simulink model "FLC_tracking_comparison_of_quadrotor"  (R2015a)
settings: Solver=ode3  StartTime=0.0  StopTime=10  FixedStep=0.01  RelTol=1e-3
libraries: simulink x9, commnoisgen2 x5, fuzblock x4
settings Model: SimulationMode=accelerator  Creator=user  LastModifiedBy=user
settings OptimizationCC: EfficientMapNaN2IntZero=off
settings HardwareCC: TargetLongLongMode=on  TargetIntDivRoundTo=Zero  TargetEndianess=LittleEndian  TargetHWDeviceType=MATLAB Host  ProdEqTarget=off
settings CodeAppCC: MaxIdLength=128
settings GRTTargetCC: CombineOutputUpdateFcns=off  GRTInterface=on

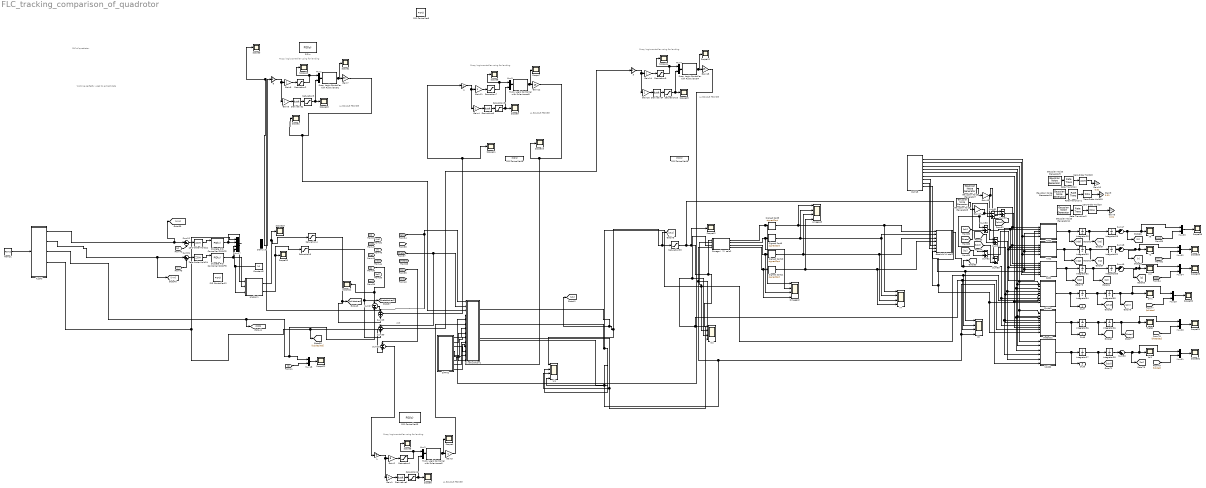
== system FLC_tracking_comparison_of_quadrotor ==
  note: Working perfectly used to extract data
  note: FLC of quadrotor
  note: d25
  note: Fuzzy logic controller using for landing
  note: LA BOUCLE FERMEE
  note: Fuzzy logic controller using for landing
  note: LA BOUCLE FERMEE
  note: Fuzzy logic controller using for landing
  note: LA BOUCLE FERMEE
  note: Fuzzy logic controller using for landing
  note: LA BOUCLE FERMEE
  1 : Gain  Gain=5
  2 : Gain
  3 : Gain
  8 : Gain  Gain=5
  Constant2 : Constant  Value=10
  DATA2 : MATLAB Function  TreatAsAtomicUnit=on
  DATA5 : MATLAB Function  TreatAsAtomicUnit=on
  Demux3 : Demux  Outputs=2
  Derivative{1..4} (4 alike) : Derivative
  Discrete PID Controller (2DOF)2 : simulink/Continuous/PID Controller (2DOF)  Controller=PID  TimeDomain=Discrete-time  SampleTime=0.01  IntegratorMethod=Forward Euler  FilterMethod=Forward Euler  Form=Parallel  UseFilter=on  ControllerParametersSource=internal  P=40  I=10  D=1  N=100  b=1  c=1  InitialConditionSource=internal  InitialConditionForIntegrator=0  InitialConditionForFilter=0  ExternalReset=none  LimitOutput=off  UpperSaturationLimit=inf  LowerSaturationLimit=-inf  LinearizeAsGain=off  AntiWindupMode=none  Kb=1  TrackingMode=off  Kt=1  PParamMin=[]  PParamMax=[]  IParamMin=[]  IParamMax=[]  DParamMin=[]  DParamMax=[]  NParamMin=[]  NParamMax=[]  bParamMin=[]  bParamMax=[]  cParamMin=[]  cParamMax=[]  KbParamMin=[]  KbParamMax=[]  KtParamMin=[]  KtParamMax=[]  POutMin=[]  POutMax=[]  IOutMin=[]  IOutMax=[]  DOutMin=[]  DOutMax=[]  NOutMin=[]  NOutMax=[]  bOutMin=[]  bOutMax=[]  cOutMin=[]  cOutMax=[]  KbOutMin=[]  KbOutMax=[]  KtOutMin=[]  KtOutMax=[]  IntegratorOutMin=[]  IntegratorOutMax=[]  FilterOutMin=[]  FilterOutMax=[]  SumOutMin=[]  SumOutMax=[]  Sum1OutMin=[]  Sum1OutMax=[]  Sum2OutMin=[]  Sum2OutMax=[]  Sum3OutMin=[]  Sum3OutMax=[]  SumI1OutMin=[]  SumI1OutMax=[]  SumI2OutMin=[]  SumI2OutMax=[]  SumI3OutMin=[]  SumI3OutMax=[]  SumDOutMin=[]  SumDOutMax=[]  SaturationOutMin=[]  SaturationOutMax=[]  IntegratorContinuousStateAttributes=''  IntegratorStateMustResolveToSignalObject=off  IntegratorRTWStateStorageClass=Auto  FilterContinuousStateAttributes=''  FilterStateMustResolveToSignalObject=off  FilterRTWStateStorageClass=Auto  DifferentiatorICPrevScaledInput=0  DifferentiatorOutMin=[]  DifferentiatorOutMax=[]
  Discrete PID Controller (2DOF)3 : simulink/Continuous/PID Controller (2DOF)  Controller=PID  TimeDomain=Discrete-time  SampleTime=0.01  IntegratorMethod=Forward Euler  FilterMethod=Forward Euler  Form=Parallel  UseFilter=on  ControllerParametersSource=internal  P=30  I=8  D=2.4  N=100  b=1  c=1  InitialConditionSource=internal  InitialConditionForIntegrator=0  InitialConditionForFilter=0  ExternalReset=none  LimitOutput=off  UpperSaturationLimit=inf  LowerSaturationLimit=-inf  LinearizeAsGain=off  AntiWindupMode=none  Kb=1  TrackingMode=off  Kt=1  PParamMin=[]  PParamMax=[]  IParamMin=[]  IParamMax=[]  DParamMin=[]  DParamMax=[]  NParamMin=[]  NParamMax=[]  bParamMin=[]  bParamMax=[]  cParamMin=[]  cParamMax=[]  KbParamMin=[]  KbParamMax=[]  KtParamMin=[]  KtParamMax=[]  POutMin=[]  POutMax=[]  IOutMin=[]  IOutMax=[]  DOutMin=[]  DOutMax=[]  NOutMin=[]  NOutMax=[]  bOutMin=[]  bOutMax=[]  cOutMin=[]  cOutMax=[]  KbOutMin=[]  KbOutMax=[]  KtOutMin=[]  KtOutMax=[]  IntegratorOutMin=[]  IntegratorOutMax=[]  FilterOutMin=[]  FilterOutMax=[]  SumOutMin=[]  SumOutMax=[]  Sum1OutMin=[]  Sum1OutMax=[]  Sum2OutMin=[]  Sum2OutMax=[]  Sum3OutMin=[]  Sum3OutMax=[]  SumI1OutMin=[]  SumI1OutMax=[]  SumI2OutMin=[]  SumI2OutMax=[]  SumI3OutMin=[]  SumI3OutMax=[]  SumDOutMin=[]  SumDOutMax=[]  SaturationOutMin=[]  SaturationOutMax=[]  IntegratorContinuousStateAttributes=''  IntegratorStateMustResolveToSignalObject=off  IntegratorRTWStateStorageClass=Auto  FilterContinuousStateAttributes=''  FilterStateMustResolveToSignalObject=off  FilterRTWStateStorageClass=Auto  DifferentiatorICPrevScaledInput=0  DifferentiatorOutMin=[]  DifferentiatorOutMax=[]
  Fuzzy Logic Controller with Ruleviewer{1..4} (4 alike) : fuzblock/Fuzzy Logic  Controller  with Ruleviewer  fismatrix=fuzzytrial7  Ts=2
  Gain1 : Gain  Gain=4
  Gain{8..10,13,17} (5 alike) : Gain  Gain=0.01
  Gain{3..6,11,14,16} (7 alike) : Gain
  Gain12 : Gain  Gain=15
  Gain15 : Gain  Gain=15
  Gain2 : Gain  Gain=8
  Gain7 : Gain  Gain=50
  Gaussian Noise Generator10 : commnoisgen2/Gaussian Noise Generator  m=0  d=1  s=41  Ts=3  frameBased=off  sampPerFrame=1  orient=off  outDataType=single
  Gaussian Noise Generator11 : commnoisgen2/Gaussian Noise Generator  m=0  d=1  s=41  Ts=4  frameBased=off  sampPerFrame=1  orient=off  outDataType=single
  Gaussian Noise Generator7 : commnoisgen2/Gaussian Noise Generator  m=0  d=1  s=41  Ts=0.01  frameBased=off  sampPerFrame=1  orient=off  outDataType=double
  Gaussian Noise Generator8 : commnoisgen2/Gaussian Noise Generator  m=0  d=1  s=41  Ts=0.01  frameBased=off  sampPerFrame=1  orient=off  outDataType=double
  Gaussian Noise Generator9 : commnoisgen2/Gaussian Noise Generator  m=0  d=1  s=41  Ts=5  frameBased=off  sampPerFrame=1  orient=off  outDataType=single
  Integrator{25..36} (12 alike) : Integrator
  Mux{1..4,18,29..34} (11 alike) : Mux  Inputs=2
  Mux17 : Mux
  Omega i ^2  calc2 : MATLAB Function  TreatAsAtomicUnit=on
  Omegas2 : Scope  NumInputPorts=4
      settings: YMin=-5~-5~-5~-5  YMax=5~5~5~5  SaveName=ScopeData36
  PID Controller12 : simulink/Continuous/PID Controller  Controller=PID  TimeDomain=Continuous-time  SampleTime=-1  IntegratorMethod=Forward Euler  FilterMethod=Forward Euler  Form=Parallel  UseFilter=on  ControllerParametersSource=internal  P=1.8  I=0.4  D=2.4  N=100  InitialConditionSource=internal  InitialConditionForIntegrator=0  InitialConditionForFilter=0  ExternalReset=none  LimitOutput=off  UpperSaturationLimit=inf  LowerSaturationLimit=-inf  LinearizeAsGain=on  AntiWindupMode=none  Kb=1  TrackingMode=off  Kt=1  PParamMin=[]  PParamMax=[]  IParamMin=[]  IParamMax=[]  DParamMin=[]  DParamMax=[]  NParamMin=[]  NParamMax=[]  KbParamMin=[]  KbParamMax=[]  KtParamMin=[]  KtParamMax=[]  POutMin=[]  POutMax=[]  IOutMin=[]  IOutMax=[]  DOutMin=[]  DOutMax=[]  NOutMin=[]  NOutMax=[]  KbOutMin=[]  KbOutMax=[]  KtOutMin=[]  KtOutMax=[]  IntegratorOutMin=[]  IntegratorOutMax=[]  FilterOutMin=[]  FilterOutMax=[]  SumOutMin=[]  SumOutMax=[]  SumI1OutMin=[]  SumI1OutMax=[]  SumI2OutMin=[]  SumI2OutMax=[]  SumI3OutMin=[]  SumI3OutMax=[]  SumDOutMin=[]  SumDOutMax=[]  SaturationOutMin=[]  SaturationOutMax=[]  IntegratorContinuousStateAttributes=''  IntegratorStateMustResolveToSignalObject=off  IntegratorRTWStateStorageClass=Auto  FilterContinuousStateAttributes=''  FilterStateMustResolveToSignalObject=off  FilterRTWStateStorageClass=Auto  DifferentiatorICPrevScaledInput=0  DifferentiatorOutMin=[]  DifferentiatorOutMax=[]
  PID Controller13 : simulink/Continuous/PID Controller  Controller=PID  TimeDomain=Continuous-time  SampleTime=-1  IntegratorMethod=Forward Euler  FilterMethod=Forward Euler  Form=Parallel  UseFilter=on  ControllerParametersSource=internal  P=4.05643234281984  I=0.70959032661118  D=4.0859309721323  N=476.409993785115  InitialConditionSource=internal  InitialConditionForIntegrator=0  InitialConditionForFilter=0  ExternalReset=none  LimitOutput=off  UpperSaturationLimit=inf  LowerSaturationLimit=-inf  LinearizeAsGain=on  AntiWindupMode=none  Kb=1  TrackingMode=off  Kt=1  PParamMin=[]  PParamMax=[]  IParamMin=[]  IParamMax=[]  DParamMin=[]  DParamMax=[]  NParamMin=[]  NParamMax=[]  KbParamMin=[]  KbParamMax=[]  KtParamMin=[]  KtParamMax=[]  POutMin=[]  POutMax=[]  IOutMin=[]  IOutMax=[]  DOutMin=[]  DOutMax=[]  NOutMin=[]  NOutMax=[]  KbOutMin=[]  KbOutMax=[]  KtOutMin=[]  KtOutMax=[]  IntegratorOutMin=[]  IntegratorOutMax=[]  FilterOutMin=[]  FilterOutMax=[]  SumOutMin=[]  SumOutMax=[]  SumI1OutMin=[]  SumI1OutMax=[]  SumI2OutMin=[]  SumI2OutMax=[]  SumI3OutMin=[]  SumI3OutMax=[]  SumDOutMin=[]  SumDOutMax=[]  SaturationOutMin=[]  SaturationOutMax=[]  IntegratorContinuousStateAttributes=''  IntegratorStateMustResolveToSignalObject=off  IntegratorRTWStateStorageClass=Auto  FilterContinuousStateAttributes=''  FilterStateMustResolveToSignalObject=off  FilterRTWStateStorageClass=Auto  DifferentiatorICPrevScaledInput=0  DifferentiatorOutMin=[]  DifferentiatorOutMax=[]
  PID Controller15 : simulink/Continuous/PID Controller  Controller=PID  TimeDomain=Continuous-time  SampleTime=-1  IntegratorMethod=Forward Euler  FilterMethod=Forward Euler  Form=Parallel  UseFilter=on  ControllerParametersSource=internal  P=11  I=0.2  D=22  N=100  InitialConditionSource=internal  InitialConditionForIntegrator=0  InitialConditionForFilter=0  ExternalReset=none  LimitOutput=off  UpperSaturationLimit=inf  LowerSaturationLimit=-inf  LinearizeAsGain=on  AntiWindupMode=none  Kb=1  TrackingMode=off  Kt=1  PParamMin=[]  PParamMax=[]  IParamMin=[]  IParamMax=[]  DParamMin=[]  DParamMax=[]  NParamMin=[]  NParamMax=[]  KbParamMin=[]  KbParamMax=[]  KtParamMin=[]  KtParamMax=[]  POutMin=[]  POutMax=[]  IOutMin=[]  IOutMax=[]  DOutMin=[]  DOutMax=[]  NOutMin=[]  NOutMax=[]  KbOutMin=[]  KbOutMax=[]  KtOutMin=[]  KtOutMax=[]  IntegratorOutMin=[]  IntegratorOutMax=[]  FilterOutMin=[]  FilterOutMax=[]  SumOutMin=[]  SumOutMax=[]  SumI1OutMin=[]  SumI1OutMax=[]  SumI2OutMin=[]  SumI2OutMax=[]  SumI3OutMin=[]  SumI3OutMax=[]  SumDOutMin=[]  SumDOutMax=[]  SaturationOutMin=[]  SaturationOutMax=[]  IntegratorContinuousStateAttributes=''  IntegratorStateMustResolveToSignalObject=off  IntegratorRTWStateStorageClass=Auto  FilterContinuousStateAttributes=''  FilterStateMustResolveToSignalObject=off  FilterRTWStateStorageClass=Auto  DifferentiatorICPrevScaledInput=0  DifferentiatorOutMin=[]  DifferentiatorOutMax=[]
  PID Controller16 : simulink/Continuous/PID Controller  Controller=PID  TimeDomain=Continuous-time  SampleTime=-1  IntegratorMethod=Forward Euler  FilterMethod=Forward Euler  Form=Parallel  UseFilter=on  ControllerParametersSource=internal  P=12  I=0.2  D=20  N=100  InitialConditionSource=internal  InitialConditionForIntegrator=0  InitialConditionForFilter=0  ExternalReset=none  LimitOutput=off  UpperSaturationLimit=inf  LowerSaturationLimit=-inf  LinearizeAsGain=on  AntiWindupMode=none  Kb=1  TrackingMode=off  Kt=1  PParamMin=[]  PParamMax=[]  IParamMin=[]  IParamMax=[]  DParamMin=[]  DParamMax=[]  NParamMin=[]  NParamMax=[]  KbParamMin=[]  KbParamMax=[]  KtParamMin=[]  KtParamMax=[]  POutMin=[]  POutMax=[]  IOutMin=[]  IOutMax=[]  DOutMin=[]  DOutMax=[]  NOutMin=[]  NOutMax=[]  KbOutMin=[]  KbOutMax=[]  KtOutMin=[]  KtOutMax=[]  IntegratorOutMin=[]  IntegratorOutMax=[]  FilterOutMin=[]  FilterOutMax=[]  SumOutMin=[]  SumOutMax=[]  SumI1OutMin=[]  SumI1OutMax=[]  SumI2OutMin=[]  SumI2OutMax=[]  SumI3OutMin=[]  SumI3OutMax=[]  SumDOutMin=[]  SumDOutMax=[]  SaturationOutMin=[]  SaturationOutMax=[]  IntegratorContinuousStateAttributes=''  IntegratorStateMustResolveToSignalObject=off  IntegratorRTWStateStorageClass=Auto  FilterContinuousStateAttributes=''  FilterStateMustResolveToSignalObject=off  FilterRTWStateStorageClass=Auto  DifferentiatorICPrevScaledInput=0  DifferentiatorOutMin=[]  DifferentiatorOutMax=[]
  PID Controller8 : simulink/Continuous/PID Controller  Controller=PID  TimeDomain=Discrete-time  SampleTime=0.01  IntegratorMethod=Forward Euler  FilterMethod=Forward Euler  Form=Parallel  UseFilter=off  ControllerParametersSource=internal  P=0.106391194484536  I=0.00161865601075222  D=1.74822294381308  N=100  InitialConditionSource=internal  InitialConditionForIntegrator=0  InitialConditionForFilter=0  ExternalReset=none  LimitOutput=off  UpperSaturationLimit=inf  LowerSaturationLimit=-inf  LinearizeAsGain=on  AntiWindupMode=none  Kb=1  TrackingMode=off  Kt=1  PParamMin=[]  PParamMax=[]  IParamMin=[]  IParamMax=[]  DParamMin=[]  DParamMax=[]  NParamMin=[]  NParamMax=[]  KbParamMin=[]  KbParamMax=[]  KtParamMin=[]  KtParamMax=[]  POutMin=[]  POutMax=[]  IOutMin=[]  IOutMax=[]  DOutMin=[]  DOutMax=[]  NOutMin=[]  NOutMax=[]  KbOutMin=[]  KbOutMax=[]  KtOutMin=[]  KtOutMax=[]  IntegratorOutMin=[]  IntegratorOutMax=[]  FilterOutMin=[]  FilterOutMax=[]  SumOutMin=[]  SumOutMax=[]  SumI1OutMin=[]  SumI1OutMax=[]  SumI2OutMin=[]  SumI2OutMax=[]  SumI3OutMin=[]  SumI3OutMax=[]  SumDOutMin=[]  SumDOutMax=[]  SaturationOutMin=[]  SaturationOutMax=[]  IntegratorContinuousStateAttributes=''  IntegratorStateMustResolveToSignalObject=off  IntegratorRTWStateStorageClass=Auto  FilterContinuousStateAttributes=''  FilterStateMustResolveToSignalObject=off  FilterRTWStateStorageClass=Auto  DifferentiatorICPrevScaledInput=0  DifferentiatorOutMin=[]  DifferentiatorOutMax=[]
  PID z : simulink/Continuous/PID Controller  Controller=PID  TimeDomain=Continuous-time  SampleTime=-1  IntegratorMethod=Forward Euler  FilterMethod=Forward Euler  Form=Parallel  UseFilter=on  ControllerParametersSource=internal  P=4  I=2  D=5  N=476.409993785115  InitialConditionSource=internal  InitialConditionForIntegrator=0  InitialConditionForFilter=0  ExternalReset=none  LimitOutput=off  UpperSaturationLimit=inf  LowerSaturationLimit=-inf  LinearizeAsGain=on  AntiWindupMode=none  Kb=1  TrackingMode=off  Kt=1  PParamMin=[]  PParamMax=[]  IParamMin=[]  IParamMax=[]  DParamMin=[]  DParamMax=[]  NParamMin=[]  NParamMax=[]  KbParamMin=[]  KbParamMax=[]  KtParamMin=[]  KtParamMax=[]  POutMin=[]  POutMax=[]  IOutMin=[]  IOutMax=[]  DOutMin=[]  DOutMax=[]  NOutMin=[]  NOutMax=[]  KbOutMin=[]  KbOutMax=[]  KtOutMin=[]  KtOutMax=[]  IntegratorOutMin=[]  IntegratorOutMax=[]  FilterOutMin=[]  FilterOutMax=[]  SumOutMin=[]  SumOutMax=[]  SumI1OutMin=[]  SumI1OutMax=[]  SumI2OutMin=[]  SumI2OutMax=[]  SumI3OutMin=[]  SumI3OutMax=[]  SumDOutMin=[]  SumDOutMax=[]  SaturationOutMin=[]  SaturationOutMax=[]  IntegratorContinuousStateAttributes=''  IntegratorStateMustResolveToSignalObject=off  IntegratorRTWStateStorageClass=Auto  FilterContinuousStateAttributes=''  FilterStateMustResolveToSignalObject=off  FilterRTWStateStorageClass=Auto  DifferentiatorICPrevScaledInput=0  DifferentiatorOutMin=[]  DifferentiatorOutMax=[]
  Phidd2 : MATLAB Function  TreatAsAtomicUnit=on
  Ramp1 : simulink/Sources/Ramp  slope=1  start=0  X0=0
  Rate Transition : RateTransition
  Rate Transition1 : RateTransition
  Rate Transition2 : RateTransition
  Saturation1 : Saturate  UpperLimit=4  LowerLimit=-4
  Saturation{3,6..10} (6 alike) : Saturate  UpperLimit=5  LowerLimit=-5
  Saturation2 : Saturate  UpperLimit=4  LowerLimit=-4
  Saturation33 : Saturate  UpperLimit=25  LowerLimit=1
  Saturation4 : Saturate  UpperLimit=0.4  LowerLimit=-0.4
  Saturation5 : Saturate  UpperLimit=0.4  LowerLimit=-0.41
  Scope{1..15,18..22,38..39,42,50..53} (27 alike) : Scope
      Scope1 settings: SaveName=ScopeData19
      Scope10 settings: SaveName=ScopeData10
      Scope11 settings: SaveName=ScopeData11
      Scope12 settings: SaveName=ScopeData15
      Scope14 settings: SaveName=ScopeData16
      Scope15 settings: SaveName=ScopeData20
      Scope19 settings: TimeRange=10  YMin=-0.314159  YMax=-0.314159  SaveName=ScopeData12
      Scope2 settings: SaveName=ScopeData2
      Scope20 settings: SaveName=ScopeData13
      Scope21 settings: SaveName=ScopeData14
      Scope22 settings: YMin=-0.025  YMax=0.015  SaveName=ScopeData17
      Scope3 settings: SaveName=ScopeData3
      Scope38 settings: TimeRange=35  YMin=-8  YMax=6  SaveName=xdata2
      Scope39 settings: YMin=7.955  YMax=7.9725  SaveName=zdata2
      Scope4 settings: SaveName=ScopeData4
      Scope42 settings: SaveName=ScopeData40
      Scope5 settings: SaveName=ScopeData5
      Scope50 settings: YMin=-0.125  YMax=0.125  SaveName=phi_ang
      Scope51 settings: YMin=-0.525  YMax=-0.275  SaveName=theta_ang
      Scope52 settings: YMin=-0.002  YMax=0  SaveName=ksi_ang
      Scope53 settings: YMin=11  YMax=28  SaveName=ydata2
      Scope6 settings: SaveName=ScopeData6
      Scope7 settings: SaveName=ScopeData7
      Scope8 settings: SaveName=ScopeData8
      Scope9 settings: SaveName=ScopeData9
  Signed Sqrt{8..11} (4 alike) : Sqrt  Operator=signedSqrt  SaturateOnIntegerOverflow=on
  Sum12 : Sum  Inputs=|+-
  Sum{27..30,51..55,58} (10 alike) : Sum  Inputs=-+
  Sum31 : Sum  Inputs=|+-
  Sum47 : Sum  Inputs=++|
  Sum48 : Sum  Inputs=++|
  Sum49 : Sum  Inputs=++|
  Sum50 : Sum  Inputs=|++
  Ui calculation1 : MATLAB Function  TreatAsAtomicUnit=on
  Ui1 : Scope  NumInputPorts=4
      settings: YMin=12.5911~0.0906136~-0.496862~0.0613624  YMax=13.9165~0.100152~-0.449542~0.0678216  SaveName=ScopeData18
  Ui2 : Scope  NumInputPorts=4
      settings: YMin=-5~-5~-5~-5  YMax=5~5~5~5  SaveName=ScopeData48
  X6 : Scope
      settings: YMin=3.81  YMax=3.95  SaveName=ScopeData49
  X7 : Scope  NumInputPorts=4
      settings: YMin=-5~-5~-5~-5  YMax=5~5~5~5  SaveName=ScopeData50
  X8 : Scope  NumInputPorts=4
      settings: YMin=-5~-5~-5~-5  YMax=5~5~5~5  SaveName=ScopeData51
  Xdd2 : MATLAB Function  TreatAsAtomicUnit=on
  Y2 : Scope
      settings: YMin=-0.01095  YMax=-0.0103  SaveName=ScopeData52
  Ydd2 : MATLAB Function  TreatAsAtomicUnit=on
  Z 2 : Scope
      settings: YMin=7.615  YMax=7.6215  SaveName=ScopeData53
  Zdd2 : MATLAB Function  TreatAsAtomicUnit=on
  Zero-Order Hold{18..20,22,24} (5 alike) : ZeroOrderHold  SampleTime=0.01
  angles 1 : MATLAB Function  TreatAsAtomicUnit=on
  "hjsdfd " : MATLAB Function  TreatAsAtomicUnit=on
  ksi1 : Scope
      settings: SaveName=ksiangle1
  ksidd2 : MATLAB Function  TreatAsAtomicUnit=on
  omegas3 : Scope  NumInputPorts=4
      settings: YMin=-5~-5~-5~-5  YMax=5~5~5~5  SaveName=ScopeData54
  phi1 : Scope
      settings: SaveName=phiangle1
  recalc of Ui real2 : MATLAB Function  TreatAsAtomicUnit=on
  theta1 : Scope
      settings: SaveName=thetaangle1
  thetadd2 : MATLAB Function  TreatAsAtomicUnit=on
  Out7 : Outport
  Out8 : Outport  Port=2
  Out9 : Outport  Port=3
  wires:
  Xdd2/1(Xdd) -> [Xdd], Integrator25/1
  Ydd2/1(Ydd) -> [Ydd], Integrator30/1
  Zdd2/1(Zdd) -> [zdd], Integrator32/1
  Phidd2/1(phidd) -> Out7/1, Integrator34/1
  Integrator34/1 -> [phid], Integrator35/1
  thetadd2/1(thetadd) -> Out8/1, Integrator36/1
  Integrator36/1 -> [thetad], Integrator26/1
  ksidd2/1(ksidd) -> Out9/1, Integrator27/1
  Integrator27/1 -> [ksid], Integrator28/1
  Integrator35/1 -> Mux29/1, phi1/1, [phi]
  DATA5/1(m) -> Zdd2/5(m), Ydd2/5(m), Xdd2/5(m)
  DATA5/2(g) -> Zdd2/6(g)
  DATA5/3(Ixx) -> ksidd2/1(Ixx), thetadd2/1(Ixx), Phidd2/1(Ixx)
  DATA5/4(Iyy) -> Phidd2/2(Iyy), ksidd2/2(Iyy), thetadd2/2(Iyy)
  DATA5/5(Izz) -> thetadd2/3(Izz), ksidd2/3(Izz), Phidd2/3(Izz)
  DATA5/6(J) -> thetadd2/7(J), Phidd2/7(J)
  Sum51/1 -> Zdd2/1(phi), Ydd2/1(phi), Xdd2/1(phi)
  Sum58/1 -> Zdd2/2(theta), Ydd2/2(theta), Xdd2/2(theta)
  Sum52/1 -> Xdd2/3(ksi), Zdd2/3(ksi), Ydd2/3(ksi)
  Sum54/1 -> Phidd2/4(thetad), ksidd2/5(thetad)
  Sum55/1 -> Phidd2/5(ksid), thetadd2/5(ksid)
  Sum53/1 -> ksidd2/4(phid), thetadd2/4(phid)
  recalc of Ui real2/1(omega) -> [omega], thetadd2/6(omega), Phidd2/6(omega)
  DATA5/7(b) -> recalc of Ui real2/5(b)
  DATA5/8(d) -> recalc of Ui real2/6(d)
  Ui calculation1/4(u4) -> Ui1/4, Ui2/4, Omega i ^2  calc2/4(u4), ksidd2/6(u4), X8/4
  Ui calculation1/3(u3) -> Ui2/3, Omega i ^2  calc2/3(u3), X8/3, thetadd2/8(u3), Ui1/3
  Ui calculation1/2(u2) -> X8/2, Phidd2/8(u2), Omega i ^2  calc2/2(u2), Ui2/2, Ui1/2
  Omega i ^2  calc2/1(om1) -> Omegas2/1, Signed Sqrt8/1
  Omega i ^2  calc2/2(om2) -> Omegas2/2, Signed Sqrt9/1
  Omega i ^2  calc2/3(om3) -> Omegas2/3, Signed Sqrt10/1
  Omega i ^2  calc2/4(om4) -> Omegas2/4, Signed Sqrt11/1
  Gain17/1 -> Sum52/1, Sum58/1, Sum51/1
  [phi] -> Sum51/2
  [theta] -> Sum58/2
  [ksi] -> Sum52/2
  Gain13/1 -> Sum55/1, Sum53/1, Sum54/1
  [phid] -> Sum53/2
  [thetad] -> Sum54/2
  [ksid] -> Sum55/2
  Saturation33/1 -> X8/1, Zdd2/4(u1), Ydd2/4(u1), Xdd2/4(u1), Scope42/1, Ui2/1, Omega i ^2  calc2/1(u1)
  Integrator32/1 -> [zd], Integrator33/1
  Integrator30/1 -> [Yd], Integrator31/1
  Integrator25/1 -> [Xd], Integrator29/1
  DATA5/9(l) -> Phidd2/9(l), thetadd2/9(l), recalc of Ui real2/7(l)
  [phides] -> Mux29/2
  Mux29/1 -> Scope50/1
  Integrator26/1 -> [theta], Mux30/1, theta1/1
  [thetades] -> Mux30/2
  Mux30/1 -> Scope51/1
  Sum50/1 -> [ksi], Mux31/1, ksi1/1
  [ksides] -> Mux31/2
  Mux31/1 -> Scope52/1
  Sum48/1 -> [Y], Mux32/1, Y2/1
  [YYY] -> Mux32/2
  Mux32/1 -> Scope53/1
  Sum47/1 -> [X], Mux33/1, X6/1
  [XXX] -> Mux33/2
  Mux33/1 -> Scope38/1
  Sum49/1 -> Mux34/1, Z 2/1, [Z]
  [ZZZ] -> Mux34/2
  Mux34/1 -> Scope39/1
  Ui calculation1/1(u1) -> Ui1/1, [U11], Saturation33/1, [U1]
  Signed Sqrt8/1 -> X7/1, recalc of Ui real2/1(om1), omegas3/1
  Signed Sqrt9/1 -> X7/2, recalc of Ui real2/2(om2), omegas3/2
  Signed Sqrt10/1 -> X7/3, recalc of Ui real2/3(om3), omegas3/3
  Signed Sqrt11/1 -> X7/4, recalc of Ui real2/4(om4), omegas3/4
  Gaussian Noise Generator7/1 -> Gain13/1
  Gaussian Noise Generator8/1 -> Gain17/1
  Integrator29/1 -> Sum47/2
  Integrator31/1 -> Sum48/2
  Integrator33/1 -> Sum49/2
  Integrator28/1 -> Sum50/1
  ? -> Sum47/1
  ? -> Sum48/1
  ? -> Sum49/1
  Zero-Order Hold20/1 -> Gain8/1
  Zero-Order Hold19/1 -> Gain9/1
  Zero-Order Hold18/1 -> Gain10/1
  Rate Transition/1 -> Zero-Order Hold18/1
  Gaussian Noise Generator9/1 -> Rate Transition/1
  Rate Transition1/1 -> Zero-Order Hold19/1
  Gaussian Noise Generator10/1 -> Rate Transition1/1
  Rate Transition2/1 -> Zero-Order Hold20/1
  Gaussian Noise Generator11/1 -> Rate Transition2/1
  angles 1/1(phitrk) -> Saturation4/1, Scope19/1
  angles 1/2(thetatrk) -> Saturation5/1, Scope20/1
  DATA2/1(m) -> Ui calculation1/7(m)
  DATA2/2(g) -> Ui calculation1/8(g)
  DATA2/6(b) -> Ui calculation1/9(b)
  DATA2/7(d) -> Ui calculation1/10(d)
  DATA2/8(l) -> Ui calculation1/11(l)
  DATA2/3(Ixx) -> Ui calculation1/12(Ixx)
  DATA2/4(Iyy) -> Ui calculation1/13(Iyy)
  DATA2/5(Izz) -> Ui calculation1/14(Izz)
  "hjsdfd "/3(Zdes) -> [ZZZ], Mux18/1, Sum27/2
  [Z] -> Scope21/1, Sum27/1
  [phi] -> Ui calculation1/1(phi), Sum29/1
  [theta] -> Ui calculation1/2(theta), Sum30/1
  Sum28/1 -> 1/1
  [ksi] -> Sum28/1
  Gain3/1 -> Ui calculation1/6(ksidd)
  Sum29/1 -> Scope11/1, 2/1
  Gain15/1 -> Ui calculation1/5(thetadd)
  Gain12/1 -> Scope10/1, Ui calculation1/4(phidd)
  Saturation4/1 -> Sum29/2, [phidesired]
  Gain7/1 -> Scope2/1, Ui calculation1/3(zdd)
  [Z] -> Mux18/2
  Mux18/1 -> Scope22/1
  "hjsdfd "/4(ksides) -> [Ksidesired], Sum28/2, Mux17/1
  Sum12/1 -> Zero-Order Hold22/1
  Sum31/1 -> Zero-Order Hold24/1
  "hjsdfd "/1(Xdes) -> [XXX], Sum12/1
  [X] -> Sum12/2
  "hjsdfd "/2(Ydes) -> Sum31/1, [YYY]
  [Y] -> Sum31/2
  Discrete PID Controller (2DOF)2/1 -> angles 1/1(Xdes), Mux17/2
  Discrete PID Controller (2DOF)3/1 -> angles 1/2(Ydes), Mux17/3
  Saturation5/1 -> [thetadesired], Sum30/2
  Constant2/1 -> angles 1/3(U1), Mux17/4
  Zero-Order Hold22/1 -> Discrete PID Controller (2DOF)2/1
  Zero-Order Hold24/1 -> Discrete PID Controller (2DOF)3/1
  Mux17/1 -> ?
  ? -> Demux3/1
  ? -> ?
  Fuzzy Logic Controller with Ruleviewer1/1 -> Scope1/1, Gain7/1
  Saturation2/1 -> Mux1/1, Scope13/1
  Mux1/1 -> Fuzzy Logic Controller with Ruleviewer1/1
  Derivative2/1 -> Saturation3/1
  Gain5/1 -> Derivative2/1
  Sum27/1 -> Scope3/1, 8/1
  Saturation3/1 -> Scope18/1, Mux1/2
  Gain6/1 -> Saturation2/1
  8/1 -> Gain5/1, Gain6/1
  Fuzzy Logic Controller with Ruleviewer2/1 -> Scope4/1, Gain3/1
  Saturation1/1 -> Mux2/1, Scope5/1
  Mux2/1 -> Fuzzy Logic Controller with Ruleviewer2/1
  Derivative1/1 -> Saturation6/1
  Gain1/1 -> Derivative1/1
  Saturation6/1 -> Scope6/1, Mux2/2
  Gain2/1 -> Saturation1/1
  1/1 -> Gain1/1, Gain2/1
  Fuzzy Logic Controller with Ruleviewer3/1 -> Scope7/1, Gain12/1
  Saturation7/1 -> Mux3/1, Scope8/1
  Mux3/1 -> Fuzzy Logic Controller with Ruleviewer3/1
  Derivative3/1 -> Saturation8/1
  Gain4/1 -> Derivative3/1
  Saturation8/1 -> Scope9/1, Mux3/2
  Gain11/1 -> Saturation7/1
  2/1 -> Gain4/1, Gain11/1
  Sum30/1 -> 3/1
  Fuzzy Logic Controller with Ruleviewer4/1 -> Scope12/1, Gain15/1
  Saturation9/1 -> Mux4/1, Scope14/1
  Mux4/1 -> Fuzzy Logic Controller with Ruleviewer4/1
  Derivative4/1 -> Saturation10/1
  Gain16/1 -> Derivative4/1
  Saturation10/1 -> Scope15/1, Mux4/2
  Gain14/1 -> Saturation9/1
  3/1 -> Gain16/1, Gain14/1
  Ramp1/1 -> "hjsdfd "/1(t)

== matlab function FLC_tracking_comparison_of_quadrotor/hjsdfd  ==
  data: t input; Xdes output; Ydes output; Zdes output; ksides output; m output
function [Xdes,Ydes,Zdes,ksides,m] = fcn(t)

A=5;a=5;
B=10;b=4;
C=8;c=5;
Xdes=A*cos(a*0.070*t);
Ydes=A*sin(a*0.07*t);
%Zdes=C*(1-exp(-2*0.070*t));
%#codegen
m=1;
%ksides=0.2*cos(0.1*time)-0.32*sin(0.2*time);
ksides=0;
%plot3(Xdes,Ydes,Zdes,'*')
%hold on
%grid on
Zdes=t;
%Xdes=(5+sin(0.3*Zdes))*sin (2*pi*t/5);
%Ydes=(7+cos(0.3*Zdes))*cos (2*pi*t/5);

== matlab function FLC_tracking_comparison_of_quadrotor/DATA2 ==
  data: m output; g output; Ixx output; Iyy output; Izz output; b output; d output; l output
function [m,g,Ixx,Iyy,Izz,b,d,l] = fcn
m=1;
g=9.81;

Ixx=1*0.008;
Iyy=1*0.008;
Izz=1*0.015;
b=0.0001;
d=0.000001;
l=0.25;
%J=0.0001;

== matlab function FLC_tracking_comparison_of_quadrotor/Ui calculation1 ==
  data: phi input; theta input; zdd input; u1 output; phidd input; thetadd input; ksidd input; u2 output; u3 output; u4 output; m input; g input; b input; d input; l input; Ixx input; Iyy input; Izz input
function [u1,u2,u3,u4] = fcn(phi, theta ,zdd, phidd, thetadd,ksidd,m,g,b,d,l,Ixx,Iyy,Izz )
%#codegen
u1=0;
u2=0;
u3=0;
u4=0;
u1= (zdd+g)*m/(cos(theta)*cos(phi));
u2= phidd*Ixx;
u3= thetadd*Iyy;
u4= ksidd*Izz;
b;
d;
l;
m;
g;

% if theta ==pi/2
%     u1=100;
% else 
%     if phi==pi/2
%         u1=100;
%     else
%             
% u1= (zdd+g)*m/(cos(theta)*cos(phi));
% u2= phidd*Ixx;
% u3= thetadd*Iyy;
% u4= ksidd*Izz;
% b;
% d;
% l;
% m;
% g;
% 
%     end
% end

== matlab function FLC_tracking_comparison_of_quadrotor/angles 1 ==
  data: Xdes input; phitrk output; Ydes input; U1 input; thetatrk output
function [phitrk,thetatrk]  = fcn(Xdes,Ydes,U1)
%#codegen
m=1;
if U1<=5
    phitrk=0;
else
    if (abs(Ydes*m/U1) >= 0.3)
        phitrk= -sign(Ydes*m/U1)*pi/10;
    else
    phitrk=-asin(Ydes*m/U1);
    end
end
%%%%%%%%%%%%%%%%%%
if U1<=5
    thetatrk=0;
elseif (abs( Xdes*m/(U1*cos(phitrk)) ) >= 0.3 )
        thetatrk = sign( Xdes*m/(U1*cos(phitrk)) )*pi/10 ;
    else
    thetatrk=asin(Xdes*m/(U1*cos(phitrk)) );
end

    
%%%%%%%%%%%%
if phitrk > pi/3
    phitrk=pi/3;
end
if phitrk < -pi/3
    phitrk=-pi/3;
end
%%%%%%%%%%%%%%%
if thetatrk > pi/3
    thetatrk=pi/3;
end
if thetatrk < -pi/3
    thetatrk=-pi/3;
end

== matlab function FLC_tracking_comparison_of_quadrotor/DATA5 ==
  data: m output; g output; Ixx output; Iyy output; Izz output; J output; b output; d output; l output
function [m,g,Ixx,Iyy,Izz,J,b,d,l] = fcn
m=1;
g=9.81;

Ixx=1*0.008;
Iyy=1*0.008;
Izz=1*0.015;
b=0.0001;
d=0.000001;
l=0.25;
J=0.0001;

== matlab function FLC_tracking_comparison_of_quadrotor/Omega i ^2  calc2 ==
  data: u1 input; om1 output; u2 input; u3 input; u4 input; om2 output; om3 output; om4 output
function [om1,om2,om3,om4] = fcn(u1,u2,u3,u4)
%#codegen
b=0.0001;
d=0.000001;
l=0.25;
A=[ 1/(4*b),0, -1/(2*b*l), -1/(4*d);1/(4*b), -1/(2*b*l),0,  1/(4*d); 1/(4*b),  0,  1/(2*b*l), -1/(4*d);1/(4*b),1/(2*b*l), 0,  1/(4*d)];
B=A*[u1;u2;u3;u4];
%[om1;om2;om3;om4]
om1= B(1);
om2=B(2);
om3=B(3);
om4=B(4);

== matlab function FLC_tracking_comparison_of_quadrotor/Phidd2 ==
  data: Ixx input; Iyy input; phidd output; Izz input; thetad input; ksid input; omega input; J input; u2 input; l input
function phidd = fcn(Ixx,Iyy,Izz,thetad, ksid,omega,J,u2,l)


phidd=1/Ixx*((Iyy-Izz)*thetad*ksid-J*thetad*omega+l*u2);

== matlab function FLC_tracking_comparison_of_quadrotor/Xdd2 ==
  data: phi input; Xdd output; theta input; ksi input; u1 input; m input
function Xdd = fcn(phi,theta, ksi,u1,m)


Xdd=(sin(ksi)*sin(phi)+cos(ksi)*sin(theta)*cos(phi))*u1/m;

== matlab function FLC_tracking_comparison_of_quadrotor/Ydd2 ==
  data: phi input; Ydd output; theta input; ksi input; u1 input; m input
function Ydd = fcn(phi,theta, ksi,u1,m)
m=1;

Ydd=(-cos(ksi)*sin(phi)+sin(ksi)*sin(theta)*cos(phi))*u1/m;

== matlab function FLC_tracking_comparison_of_quadrotor/Zdd2 ==
  data: phi input; Zdd output; theta input; ksi input; u1 input; m input; g input
function Zdd = fcn(phi,theta, ksi,u1,m,g)
m=1;
g=9.81;

Zdd=-g+(cos(theta)*cos(phi))*u1/m;

== matlab function FLC_tracking_comparison_of_quadrotor/ksidd2 ==
  data: Ixx input; Iyy input; ksidd output; Izz input; phid input; thetad input; u4 input
function ksidd = fcn(Ixx,Iyy,Izz,phid, thetad,u4)


ksidd=1/Izz*((Ixx-Iyy)*phid*thetad+u4);

== matlab function FLC_tracking_comparison_of_quadrotor/recalc of Ui real2 ==
  data: om1 input; omega output; om2 input; om3 input; om4 input; b input; d input; l input; u1 output; u2 output; u3 output; u4 output
function [omega, u1,u2,u3,u4] = fcn(om1,om2,om3,om4,b,d,l)

l=l;
omega=-om1+om2-om3+om4;
u1=b*(om1^2+om2^2+om3^2+om4^2);
u2=b*(om4^2-om2^2);
u3=b*(om3^2-om1^2);
u4=d*(om4^2+om2^2-om1^2-om3^2);

== matlab function FLC_tracking_comparison_of_quadrotor/thetadd2 ==
  data: Ixx input; Iyy input; thetadd output; Izz input; phid input; ksid input; omega input; J input; u3 input; l input
function thetadd = fcn(Ixx,Iyy,Izz,phid, ksid,omega,J,u3,l)


thetadd=1/Iyy*((Izz-Ixx)*phid*ksid+J*phid*omega+l*u3);
